simulink model "segbot3state"  (R2019b)
settings: Solver=VariableStepAuto  StartTime=0.0  StopTime=10  RelTol=1e-6
values from neighbouring files (symbols this model uses):
  alpha = (n*K_t)/R_m    (= 0.0473841554559)    [equations.m]
  beta = ((n*K_t*K_b)/R_m) + f_m    (= 0.0243757847534)    [equations.m]
  f_m = 0.0022    [equations.m]
  g = 9.81    [equations.m]
  J_m = 1e-5    (= 1e-05)    [equations.m]
  J_psi = (M*L^2)/3    (= 0.0010368)    [equations.m]
  J_w = (m*R^2)/2    (= 2.4e-05)    [equations.m]
  K3 = place(A3, B3, [-241.1937  -10  -6.5199])    [equations.m]
  K_b = 0.468    [equations.m]
  K_t = 0.317    [equations.m]
  L = 0.144/2    (= 0.072)    [equations.m]
  m = 0.03    [equations.m]
  M = 0.6    [equations.m]
  n = 1    [equations.m]
  R = 0.04    [equations.m]
  R_m = 6.69    [equations.m]
settings Model: Creator=d-blo  LastModifiedBy=Jamie
settings DataIOCC: ReturnWorkspaceOutputs=off
settings DebuggingCC: ArithmeticOperatorsInVariantConditions=warning
settings SFSimCC: CustomCodeUndefinedFunction=UseInterfaceOnly

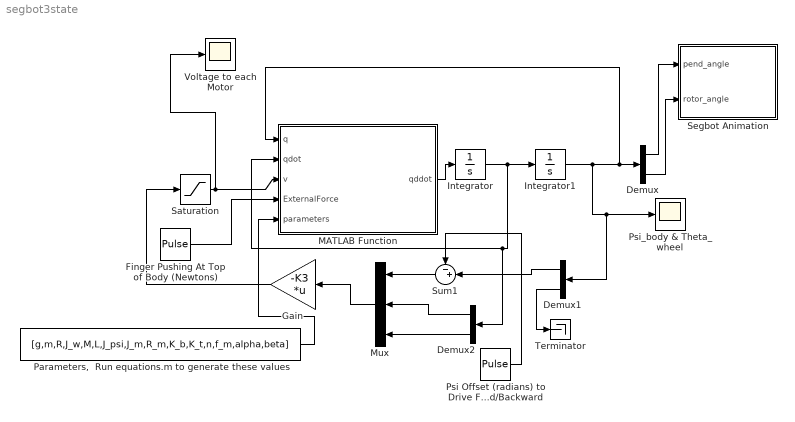
== system segbot3state ==
  Demux : Demux  Outputs=2
  Demux1 : Demux  Outputs=2
  Demux2 : Demux  Outputs=2
  Finger Pushing At Top of Body (Newtons) : DiscretePulseGenerator  PulseType=Time based  Amplitude=0.4  Period=4  PulseWidth=50  PhaseDelay=2
  Gain : Gain  Gain=-K3  Multiplication=Matrix(K*u)
  Integrator : Integrator  InitialCondition=[0 0]
  Integrator1 : Integrator  InitialCondition=[0.1 0]
  MATLAB Function : MATLAB Function  TreatAsAtomicUnit=on
  Mux : Mux  Inputs=3
  "Parameters,  Run equations.m to generate these values" : Constant  Value=[g,m,R,J_w,M,L,J_psi,J_m,R_m,K_b,K_t,n,f_m,alpha,beta]
  Psi Offset (radians) to Drive Forward/Backward : DiscretePulseGenerator  PulseType=Time based  Amplitude=0  Period=4  PulseWidth=50  PhaseDelay=2
  Psi_body & Theta_wheel : Scope
  Saturation : Saturate  UpperLimit=12.5  LowerLimit=-12.5
  Segbot Animation : Subsystem  mask(Segbot Animation){}
      mask help: The animation block takes as input the Segbot body angle (in radians), with 0 straight up and the wheel angle in radians. Use this to visualize the Segbot.
      mask Help: The animation block takes as input the Segbot body angle (in radians), with 0 straight up and the wheel angle in radians.  Use this to visualize the Segbot.
      mask Display:
      | port_label('input', 1, 'Boby Psi')
      | port_label('input', 2, 'Motor Theta')
      | fprintf('Segbot Animation')
  Sum1 : Sum  Inputs=-+|
  Terminator : Terminator
  Voltage to each Motor : Scope
  wires:
  MATLAB Function/1(qddot) -> Integrator/1
  Integrator/1 -> Demux2/1, MATLAB Function/2(qdot), Integrator1/1
  Integrator1/1 -> Demux1/1, Psi_body & Theta_wheel/1, Demux/1, MATLAB Function/1(q)
  Mux/1 -> Gain/1
  Demux/1 -> Segbot Animation/1(pend_angle)
  Demux/2 -> Segbot Animation/2(rotor_angle)
  Demux2/1 -> Mux/2
  Demux2/2 -> Mux/3
  Demux1/2 -> Terminator/1
  Gain/1 -> Saturation/1
  Saturation/1 -> Voltage to each Motor/1, MATLAB Function/3(v)
  Demux1/1 -> Sum1/2
  Psi Offset (radians) to Drive Forward/Backward/1 -> Sum1/1
  Sum1/1 -> Mux/1
  "Parameters,  Run equations.m to generate these values"/1 -> MATLAB Function/5(parameters)
  Finger Pushing At Top of Body (Newtons)/1 -> MATLAB Function/4(ExternalForce)

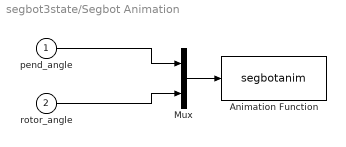
== system segbot3state/Segbot Animation ==
  pend_angle : Inport
  rotor_angle : Inport  Port=2
  Animation Function : S-Function  FunctionName=segbotanim  Parameters=0.05  SFunctionDeploymentMode=off  EnableBusSupport=off
      settings: DeleteFcn=if ~isempty(findobj('type','figure','name','dblpend1 Animation'));close('dblpend1 Animation'); end;
  Mux : Mux  Inputs=2
  wires:
  Mux/1 -> Animation Function/1
  rotor_angle/1 -> Mux/2
  pend_angle/1 -> Mux/1

== matlab function segbot3state/MATLAB Function ==
  data: q input; qddot output; qdot input; v input; ExternalForce input; parameters input
function qddot = fcn(q,qdot,v,ExternalForce,parameters)

% These are the parameters for the Lego NXTway.
% g = 9.81;
% m = 0.03;
% R = 0.04;
% J_w = (m*R^2)/2;
% M = 0.6;
% L = 0.144/2;
% J_psi = (M*L^2)/3;
% J_m = 1e-5;
% R_m = 6.69;
% K_b = 0.468;
% K_t = 0.317;
% n = 1;
% f_m = 0.0022;
% alpha = (n*K_t)/R_m;
% beta = ((n*K_t*K_b)/R_m) + f_m;

% input parameters so that you can change them in the Matlab command window
% and then they are used in your simulation.
g = parameters(1);
m = parameters(2);
R = parameters(3);
J_w = parameters(4);
M = parameters(5);
L = parameters(6);
J_psi = parameters(7);
J_m = parameters(8);
R_m = parameters(9);
K_b = parameters(10);
K_t = parameters(11);
n = parameters(12);
f_m = parameters(13);
alpha = parameters(14);
beta = parameters(15);

D = [(M*L^2 + J_psi + 2*n^2*J_m) (M*L*R*cos(q(1)) - 2*n^2*J_m);
    (M*L*R*cos(q(1)) - 2*n^2*J_m) ((2*m+M)*R^2 + 2*J_w + 2*n^2*J_m)];

h = [M*g*L*sin(q(1)) - 2*beta*qdot(1) + 2*beta*qdot(2) - 2*alpha*v + ExternalForce*L*2;
    M*L*R*(qdot(1)^2)*sin(q(1)) + 2*beta*qdot(1) - 2*beta*qdot(2) + 2*alpha*v];

qddot = inv(D)*h;
